simulink model "mdMod"  (R2013b)
settings: Solver=ode45  StartTime=0.0  StopTime=10.0  RelTol=1e-3
libraries: simulink x1
settings Model: Creator=Think79

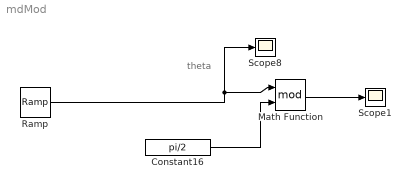
== system mdMod ==
  note: theta
  Constant16 : Constant  Value=pi/2
  Math Function : Math  Operator=mod  SaturateOnIntegerOverflow=on
  Ramp : simulink/Sources/Ramp  slope=1  start=0  X0=0
  Scope1 : Scope
  Scope8 : Scope
  wires:
  Ramp/1 -> Scope8/1, Math Function/1
  Constant16/1 -> Math Function/2
  Math Function/1 -> Scope1/1
